simulink model "LQR_Regler"  (R2019b)
settings: Solver=VariableStepAuto  StartTime=0.0  StopTime=10.0  RelTol=1e-3
undefined symbols (not defined in the file or in its folder): K_LQI
libraries: simulink x4
settings Model: Creator=qinjiaqi  LastModifiedBy=qinjiaqi

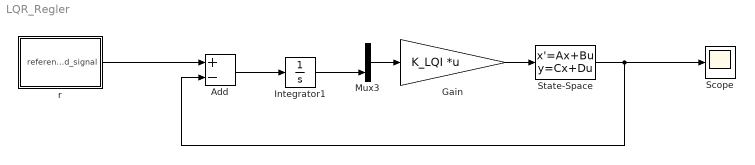
== system LQR_Regler ==
  Add : Sum  Inputs=+-
  Gain : Gain  Gain=K_LQI  Multiplication=Matrix(K*u) (u vector)
  Integrator1 : Integrator
  Mux3 : Mux  Inputs=2
  Scope : Scope
  State-Space : StateSpace  InitialCondition=0
  "r " : Subsystem
  wires:
  Add/1 -> Integrator1/1
  Gain/1 -> State-Space/1
  State-Space/1 -> Add/2, Scope/1
  "r "/1(referenced_signal) -> Add/1
  Integrator1/1 -> Mux3/2
  Mux3/1 -> Gain/1

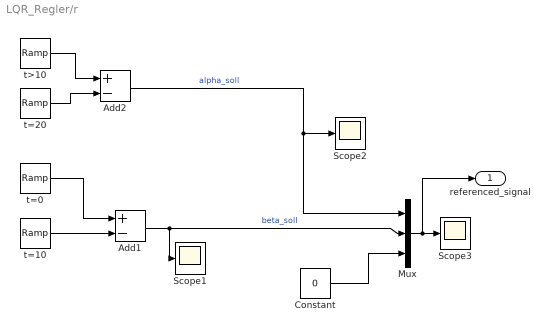
== system LQR_Regler/r  ==
  Add1 : Sum  Inputs=+-
  Add2 : Sum  Inputs=+-
  Constant : Constant  Value=0
  Mux : Mux  Inputs=3
  Scope1 : Scope
  Scope2 : Scope
  Scope3 : Scope
  t=0 : simulink/Sources/Ramp  slope=27*pi/(5*180)  start=0  InitialOutput=-27*pi/180
  t=10 : simulink/Sources/Ramp  slope=27*pi/(5*180)  start=5  InitialOutput=0
  t=20 : simulink/Sources/Ramp  slope=90*pi/(5*180)  start=15  InitialOutput=0
  t>10 : simulink/Sources/Ramp  slope=90*pi/(5*180)  start=10  InitialOutput=0
  referenced_signal : Outport
  wires:
  Mux/1 -> referenced_signal/1, Scope3/1
  t=20/1 -> Add2/2
  t=10/1 -> Add1/2
  Add1/1 -> Mux/2, Scope1/1  "beta_soll"
  t>10/1 -> Add2/1
  Add2/1 -> Mux/1, Scope2/1  "alpha_soll"
  Constant/1 -> Mux/3
  t=0/1 -> Add1/1
